simulink library "lab310_library"  (R2024b)
settings: Solver=VariableStepAuto  StartTime=0.0  StopTime=10.0  RelTol=1e-3
settings Model: Creator=micha  LastModifiedBy=micha
settings SolverCC: AlgebraicLoopSolver=TrustRegion
settings DebuggingCC: UnconnectedInputMsg=warning  UnconnectedOutputMsg=warning  UnconnectedLineMsg=warning
settings ModelReferenceCC: EnableRefExpFcnMdlSchedulingChecks=on
settings RTWCC: GPUComputeCapability=3.5  DLArmComputeVersion=19.05

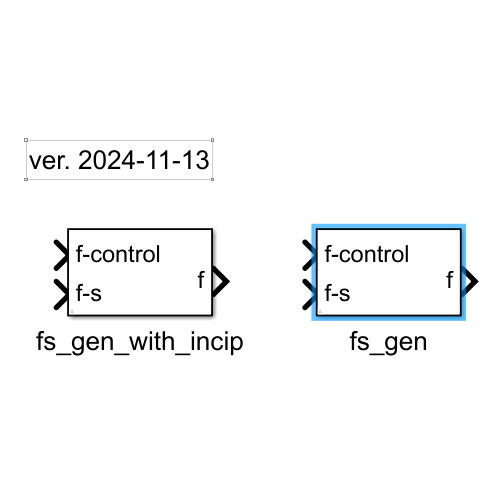
[thumbnail: Simulink's stored preview of the top-level diagram]
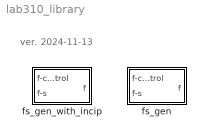
== system lab310_library ==
  note: ver. 2024-11-13
  fs_gen : Subsystem  mask{p=1, t=0}
      mask prompts: p "Czy symulujemy?"; t "Czas startu"
  fs_gen_with_incip : Subsystem  mask{p=1, t=0, st=300}
      mask prompts: p "Czy symulujemy?"; t "Czas startu"; st "Czas narastania"

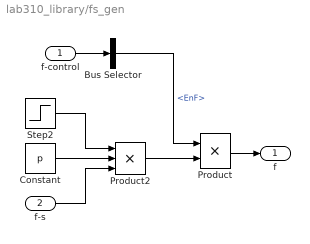
== system lab310_library/fs_gen ==
  f-control : Inport
  f-s : Inport  Port=2
  Bus Selector : BusSelector  OutputSignals=EnF
  Constant : Constant  Value=p
  Product : Product
  Product2 : Product  Inputs=3
  Step2 : Step  Time=t  SampleTime=0
  f : Outport  VectorParamsAs1DForOutWhenUnconnected=off
  wires:
  f-control/1 -> Bus Selector/1
  Product/1 -> f/1
  Bus Selector/1 -> Product/1  "<EnF>"
  f-s/1 -> Product2/3
  Step2/1 -> Product2/1
  Constant/1 -> Product2/2
  Product2/1 -> Product/2

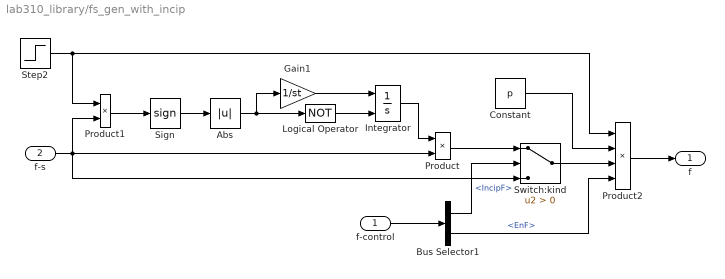
== system lab310_library/fs_gen_with_incip ==
  f-control : Inport
  f-s : Inport  Port=2
  Abs : Abs  SaturateOnIntegerOverflow=off
  Bus Selector1 : BusSelector  OutputSignals=IncipF,EnF
  Constant : Constant  Value=p
  Gain1 : Gain  Gain=1/st
  Integrator : Integrator  ExternalReset=level hold  LimitOutput=on  UpperSaturationLimit=1  LowerSaturationLimit=0
  Logical Operator : Logic  Operator=NOT  AllPortsSameDT=off  OutDataTypeStr=boolean
  Product : Product
  Product1 : Product
  Product2 : Product  Inputs=4
  Sign : Signum
  Step2 : Step  Time=t  SampleTime=0
  Switch:kind : Switch  Criteria=u2 > Threshold  SaturateOnIntegerOverflow=off  InputSameDT=off
  f : Outport  VectorParamsAs1DForOutWhenUnconnected=off
  wires:
  f-s/1 -> Product1/2, Switch:kind/3, Product/2
  Sign/1 -> Abs/1
  Logical Operator/1 -> Integrator/2
  Gain1/1 -> Integrator/1
  Abs/1 -> Gain1/1, Logical Operator/1
  f-control/1 -> Bus Selector1/1
  Bus Selector1/1 -> Switch:kind/2  "<IncipF>"
  Integrator/1 -> Product/1
  Product/1 -> Switch:kind/1
  Switch:kind/1 -> Product2/3
  Constant/1 -> Product2/2
  Step2/1 -> Product1/1, Product2/1
  Bus Selector1/2 -> Product2/4  "<EnF>"
  Product2/1 -> f/1
  Product1/1 -> Sign/1
